simulink model "static_compensator"  (R2024b)
settings: Solver=ode3  StartTime=0.0  StopTime=10  RelTol=1e-3  EnableMultiTasking=on
libraries: arduinolib x2
settings Model: ExtModeTrigDuration=2  Creator=gcampa  LastModifiedBy=Anhad Mehrotra
settings SolverCC: AlgebraicLoopSolver=TrustRegion  AutoInsertRateTranBlk=on
settings DataIOCC: LimitDataPoints=on  SaveFormat=Array  SignalLoggingSaveFormat=ModelDataLogs  ReturnWorkspaceOutputs=off
settings OptimizationCC: EnhancedBackFolding=on  PassReuseOutputArgsAs=Individual arguments  ZeroExternalMemoryAtStartup=off  ZeroInternalMemoryAtStartup=off  MaxStackSize=64  OptimizeBlockOrder=speed  DifferentSizesBufferReuse=on  OptimizationCustomize=off  EfficientTunableParamExpr=on
settings DebuggingCC: UnderspecifiedInitializationDetection=Classic  MergeDetectMultiDrivingBlocksExec=none  MultiTaskDSMMsg=warning  MultiTaskCondExecSysMsg=none  ParameterTunabilityLossMsg=error  UnconnectedInputMsg=warning  UnconnectedOutputMsg=warning  UnconnectedLineMsg=warning  SFUnexpectedBacktrackingDiag=warning  SFNoUnconditionalDefaultTransitionDiag=warning  SFExecutionAtInitializationDiag=none  ArithmeticOperatorsInVariantConditions=warning
settings HardwareCC: ProdBitPerInt=16  ProdBitPerPointer=16  ProdBitPerSizeT=16  ProdBitPerPtrDiffT=16  ProdLargestAtomicFloat=None  ProdWordSize=8  ProdHWDeviceType=Atmel->AVR  UseEmbeddedCoderFeatures=off  UseSimulinkCoderFeatures=off
settings ModelReferenceCC: PropagateSignalLabelsOutOfModel=off
settings SFSimCC: SimUseLocalCustomCode=off  MATLABDynamicMemAlloc=off  CustomCodeUndefinedFunction=UseInterfaceOnly
settings RTWCC: Description=Embedded Coder  SystemTargetFile=ert.tlc  HardwareBoard=Arduino Uno  TemplateMakefile=ert_default_tmf  RTWVerbose=off  RTWUseLocalCustomCode=off  Toolchain=Arduino AVR  BuildConfiguration=Faster Runs  GPUComputeCapability=3.5
settings CodeAppCC: ForceParamTrailComments=on  IgnoreCustomStorageClasses=off  OperatorAnnotations=on  SimulinkDataObjDesc=on  SFDataObjDesc=on  InsertBlockDesc=on
settings ERTTargetCC: SupportContinuousTime=on  SupportNonInlinedSFcns=on  SupportVariableSizeSignals=on  ExtModeTransport=3  ExtModeStaticAlloc=on  ExtModeAutomaticAllocSize=off  ExtModeStaticAllocSize=250  ExtModeMexFile=ext_xcp  ExtModeIntrfLevel=Level2 - Open  InlinedParameterPlacement=Hierarchical
settings ConfigComp: CovMetricSettings=dw  CovSaveCumulativeToWorkspaceVar=on  CovSaveSingleToWorkspaceVar=on  CovExternalEMLEnable=off

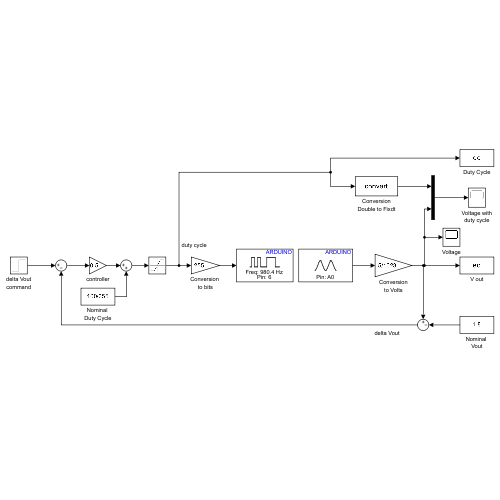
[thumbnail: Simulink's stored preview of the top-level diagram]
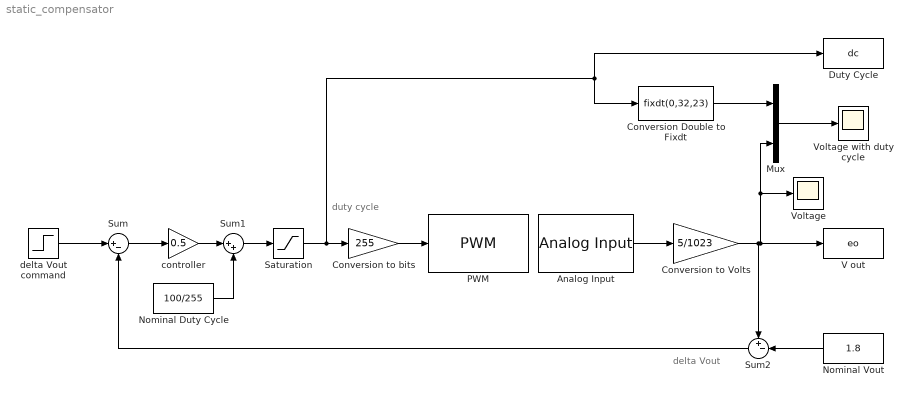
== system static_compensator ==
  note: delta Vout
  note: duty cycle
  Analog Input : arduinolib/Analog Input  pinNumber=0  ReadResultsOnly=off  ConversionTriggerSource=Software  ExternalTriggerType=uint32( 0 )  OutputDataType=uint16  EnableConversionCompleteNotify=off  EnableOuputStatus=off  SampleTime=-1  blockPlatform=arduino
  Conversion Double to Fixdt : DataTypeConversion  OutDataTypeStr=fixdt(0,32,23)  SaturateOnIntegerOverflow=off  RndMeth=Floor
  Conversion to Volts : Gain  Gain=5/1023
  Conversion to bits : Gain  Gain=255
  Duty Cycle : ToWorkspace  VariableName=dc  SaveFormat=Timeseries  SampleTime=-1
  Mux : Mux  Inputs=2
  Nominal Duty Cycle : Constant  Value=100/255
  Nominal Vout : Constant  Value=1.8
  PWM : arduinolib/PWM  pinNumber=6  frequencyType=Specify  desiredFrequency=980.4  achievableFrequency=980.4
  Saturation : Saturate  UpperLimit=1  LowerLimit=0
  Sum : Sum  Inputs=|+-
  Sum1 : Sum  Inputs=|++
  Sum2 : Sum  Inputs=+-|
  V out : ToWorkspace  VariableName=eo  SaveFormat=Timeseries  SampleTime=-1
  Voltage : Scope
  Voltage with duty cycle : Scope
  controller : Gain  Gain=0.5
  delta Vout command : Step  Time=3  SampleTime=0.02
  wires:
  Analog Input/1 -> Conversion to Volts/1
  Mux/1 -> Voltage with duty cycle/1
  Conversion to Volts/1 -> V out/1, Voltage/1, Mux/2, Sum2/1
  delta Vout command/1 -> Sum/1
  Saturation/1 -> Conversion Double to Fixdt/1, Duty Cycle/1, Conversion to bits/1
  Conversion to bits/1 -> PWM/1
  controller/1 -> Sum1/1
  Sum1/1 -> Saturation/1
  Nominal Duty Cycle/1 -> Sum1/2
  Sum2/1 -> Sum/2
  Nominal Vout/1 -> Sum2/2
  Sum/1 -> controller/1
  Conversion Double to Fixdt/1 -> Mux/1
